simulink library "variableFlow_ul"  (R2018b)
settings: Solver=VariableStepAuto  StartTime=0.0  StopTime=10.0  RelTol=1e-3
undefined symbols (not defined in the file or in its folder): env
settings Model: Creator=mcobb  LastModifiedBy=James Reed

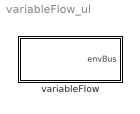
== system variableFlow_ul ==
  variableFlow : Subsystem  VariantControl=VSS_environment_constantUniformFlow

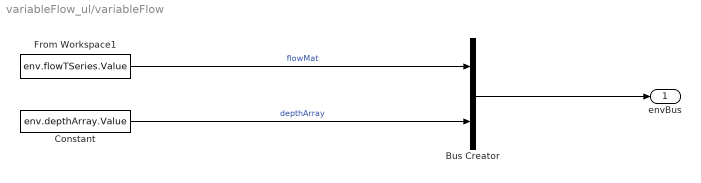
== system variableFlow_ul/variableFlow ==
  Bus Creator : BusCreator  Inputs=2  OutDataTypeStr=Bus: envBus
  Constant : Constant  Value=env.depthArray.Value
  From Workspace1 : FromWorkspace  VariableName=env.flowTSeries.Value  SampleTime=0
  envBus : Outport  OutDataTypeStr=Bus: envBus
  wires:
  Bus Creator/1 -> envBus/1
  From Workspace1/1 -> Bus Creator/1  "flowMat"
  Constant/1 -> Bus Creator/2  "depthArray"
